simulink model "eps_tno_interface_concept"  (R2016b)
settings: Solver=FixedStepAuto  StartTime=0.0  StopTime=inf  FixedStep=0.02  RelTol=1e-3
PostLoadFcn:
  | , if any(exist('dsrtsu_mdlpostloadfcn', 'file') == [2, 3, 6]), try dsrtsu_mdlpostloadfcn('Execute', bdroot); catch fprintf('Error in PostLoadFcn (dsrtsu_mdlpostloadfcn) for model "%s":\n %s\n', bdroot, lasterr); end, end,
libraries: rtican x8, simulink x8, AlgoLib x4
(part 2 of 2)

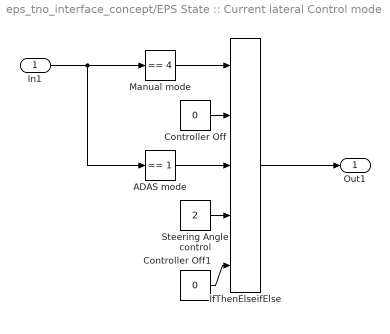
== system eps_tno_interface_concept/EPS State :: Current lateral Control mode ==
  In1 : Inport
  ADAS mode : simulink/Logic and Bit Operations/Compare To Constant  relop===  const=1  OutDataTypeStr=boolean
  Controller Off : Constant  Value=0
  Controller Off1 : Constant  Value=0
  IfThenElseifElse : AlgoLib/Signals/IfThenElseifElse
  Manual mode : simulink/Logic and Bit Operations/Compare To Constant  relop===  const=4  OutDataTypeStr=boolean
  Steering Angle control : Constant  Value=2
  Out1 : Outport
  wires:
  Controller Off1/1 -> IfThenElseifElse/5
  IfThenElseifElse/1 -> Out1/1
  Manual mode/1 -> IfThenElseifElse/1
  Controller Off/1 -> IfThenElseifElse/2
  In1/1 -> ADAS mode/1, Manual mode/1
  Steering Angle control/1 -> IfThenElseifElse/4
  ADAS mode/1 -> IfThenElseifElse/3

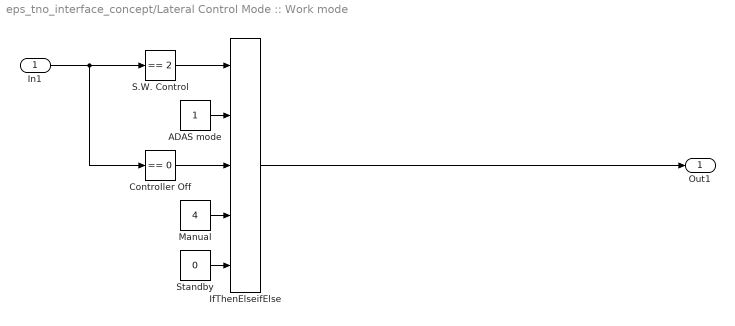
== system eps_tno_interface_concept/Lateral Control Mode :: Work mode  ==
  In1 : Inport
  ADAS mode : Constant
  Controller Off : simulink/Logic and Bit Operations/Compare To Constant  relop===  const=0  OutDataTypeStr=boolean
  IfThenElseifElse : AlgoLib/Signals/IfThenElseifElse
  Manual : Constant  Value=4
  S.W. Control : simulink/Logic and Bit Operations/Compare To Constant  relop===  const=2  OutDataTypeStr=boolean
  Standby : Constant  Value=0
  Out1 : Outport
  wires:
  Standby/1 -> IfThenElseifElse/5
  IfThenElseifElse/1 -> Out1/1
  S.W. Control/1 -> IfThenElseifElse/1
  ADAS mode/1 -> IfThenElseifElse/2
  In1/1 -> Controller Off/1, S.W. Control/1
  Manual/1 -> IfThenElseifElse/4
  Controller Off/1 -> IfThenElseifElse/3

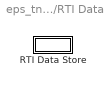
== system eps_tno_interface_concept/RTI Data ==
  RTI Data Store : Subsystem  Tag="struct('private',struct('version',struct('dsVer',uint32(2),'dsVerCreation',uint32(2),'RTI',struct('ver','7.7','type','RTI1401')),'access',struct('type','Model','isPerm',1,'created',['14-Feb-2018 14:53:06'],'modified',['03-Apr-2018 09:58:53'],'location','')),'public',struct('main',struct('data',[]),'sub',struct('name',{{'eps_tno_interfrace_concept'}},'data',{{struct('TH',struct('thTaskInfo',struct('taskType',{'TIMER','HWINT','TMRINT','SWINT','GLINT'},'tasksNumOf',{1,0,0,0,0},'srcIds',{{'TIMERA'},{},{},{},{}},'taskNames',{{['Timer Task 1']},{},{},{},{}})),'th_tc',struct('dataType','TASK','taskGroupId','','taskGroupList',{{}},'taskSchedulingPolicy','FCFS','taskType','TIMER','blkh',-1,'srcId','TIMERA','srcSgnName',['Timer A interrupt'],'srcCpuName','','taskName',['Timer Task 1  [0.02] s'],'taskNameDisplayExt','','smplTime',0.02,'smplTimeOffs',0,'hasFixedPriority',0,'priority',1,'hasFixedOvc',0,'ovcType',1,'ovcMax',1),'tc_th',struct('dataType','TASK','taskGroupId','','taskGroupList',{{}},'taskSchedulingPolicy','FCFS','taskType','TIMER','blkh',-1,'srcId','TIMERA','srcSgnName',['Timer A interrupt'],'srcCpuName','','taskName',['Timer Task 1  [0.02] s'],'taskNameDisplayExt','','smplTime',0.02,'smplTimeOffs',0,'hasFixedPriority',0,'priority',1,'hasFixedOvc',0,'ovcType',1,'ovcMax',1))}})))"  mask(RTI_DATA_STORE){}
      mask help:
      | RTI Data Store Block. This block is used by RTI to store internal model dependent data. Deleting this block will result in data loss.
      |
      | NEVER DELETE, COPY, OR MODIFY THIS BLOCK!
      mask Help:
      | RTI Data Store Block. This block is used by RTI to store internal model dependent data. Deleting this block will result in data loss.
      | 
      | NEVER DELETE, COPY, OR MODIFY THIS BLOCK!
      mask Display: text(0.5, 0.5, ' ', 'HorizontalAlignment', 'center');

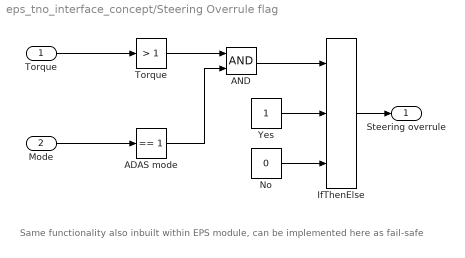
== system eps_tno_interface_concept/Steering Overrule flag ==
  note: Same functionality also inbuilt within EPS module, can be implemented here as fail-safe
  Torque : Inport
  Mode : Inport  Port=2
  ADAS mode : simulink/Logic and Bit Operations/Compare To Constant  relop===  const=1  OutDataTypeStr=boolean
  AND : Logic
  IfThenElse : AlgoLib/Signals/IfThenElse
  No : Constant  Value=0  OutDataTypeStr=boolean
  "Torque " : simulink/Logic and Bit Operations/Compare To Constant  relop=>  const=1  OutDataTypeStr=boolean
  Yes : Constant  OutDataTypeStr=boolean
  Steering overrule : Outport
  wires:
  No/1 -> IfThenElse/3
  Yes/1 -> IfThenElse/2
  Torque/1 -> "Torque "/1
  Mode/1 -> ADAS mode/1
  "Torque "/1 -> AND/1
  ADAS mode/1 -> AND/2
  AND/1 -> IfThenElse/1
  IfThenElse/1 -> Steering overrule/1

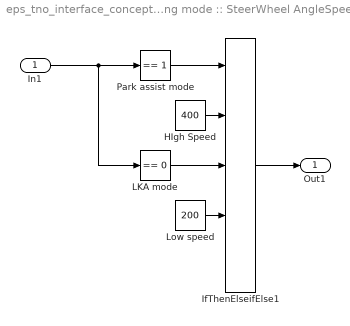
== system eps_tno_interface_concept/Steering mode :: SteerWheel AngleSpeed_ref ==
  In1 : Inport
  HIgh Speed : Constant  Value=400
  IfThenElseifElse1 : AlgoLib/Signals/IfThenElseifElse
  LKA mode : simulink/Logic and Bit Operations/Compare To Constant  relop===  const=0  OutDataTypeStr=boolean
  Low speed : Constant  Value=200
  Park assist mode : simulink/Logic and Bit Operations/Compare To Constant  relop===  const=1  OutDataTypeStr=boolean
  Out1 : Outport
  wires:
  HIgh Speed/1 -> IfThenElseifElse1/2
  Low speed/1 -> IfThenElseifElse1/4
  Park assist mode/1 -> IfThenElseifElse1/1
  LKA mode/1 -> IfThenElseifElse1/3
  IfThenElseifElse1/1 -> Out1/1
  In1/1 -> LKA mode/1, Park assist mode/1

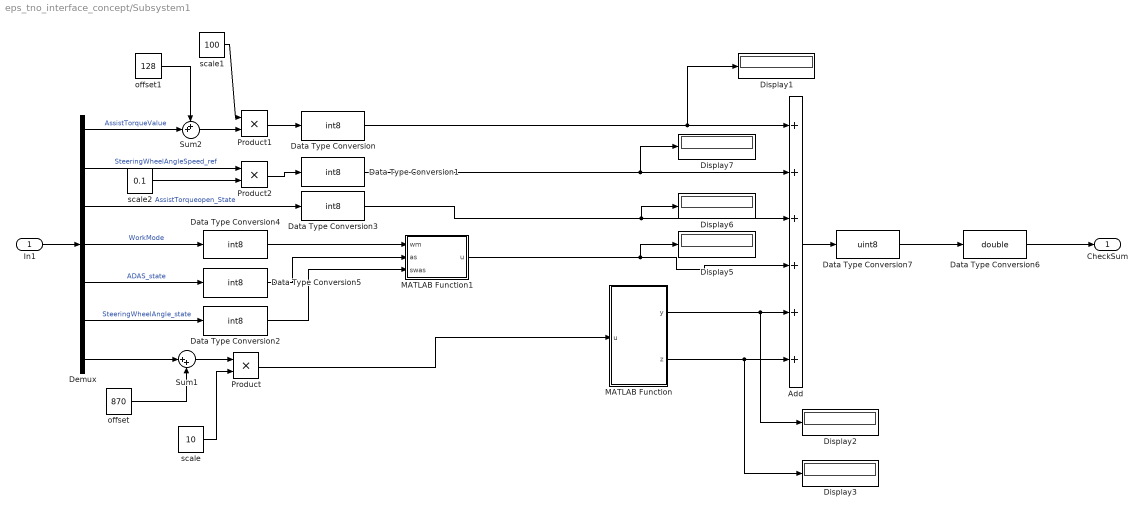
== system eps_tno_interface_concept/Subsystem1 ==
  In1 : Inport
  Add : Sum  Inputs=++++++
  Data Type Conversion{,1..5} (6 alike) : DataTypeConversion  OutDataTypeStr=int8
  Data Type Conversion6 : DataTypeConversion  OutDataTypeStr=double
  Data Type Conversion7 : DataTypeConversion  OutDataTypeStr=uint8
  Demux : Demux  Outputs=7
  Display{1..3,5..7} (6 alike) : Display
  MATLAB Function : MATLAB Function  TreatAsAtomicUnit=on
  MATLAB Function1 : MATLAB Function  TreatAsAtomicUnit=on
  Product : Product
  Product1 : Product
  Product2 : Product
  Sum1 : Sum  Inputs=|++
  Sum2 : Sum  Inputs=++|
  offset : Constant  Value=870
  offset1 : Constant  Value=128
  scale : Constant  Value=10
  scale1 : Constant  Value=100
  scale2 : Constant  Value=0.1
  CheckSum : Outport
  wires:
  In1/1 -> Demux/1
  Demux/2 -> Product2/1  "SteeringWheelAngleSpeed_ref"
  Demux/6 -> Data Type Conversion2/1  "SteeringWheelAngle_state"
  Demux/5 -> Data Type Conversion5/1  "ADAS_state"
  Demux/4 -> Data Type Conversion4/1  "WorkMode"
  Demux/3 -> Data Type Conversion3/1  "AssistTorqueopen_State"
  Data Type Conversion/1 -> Display1/1, Add/1
  Data Type Conversion1/1 -> Display7/1, Add/2
  Data Type Conversion3/1 -> Display6/1, Add/3
  Product/1 -> MATLAB Function/1(u)
  MATLAB Function/1(y) -> Display2/1, Add/5
  Data Type Conversion4/1 -> MATLAB Function1/1(wm)
  Data Type Conversion5/1 -> MATLAB Function1/2(as)
  Data Type Conversion2/1 -> MATLAB Function1/3(swas)
  MATLAB Function1/1(u) -> Display5/1, Add/4
  MATLAB Function/2(z) -> Display3/1, Add/6
  Add/1 -> Data Type Conversion7/1
  scale/1 -> Product/2
  Sum1/1 -> Product/1
  offset/1 -> Sum1/2
  Demux/7 -> Sum1/1
  Product1/1 -> Data Type Conversion/1
  Demux/1 -> Sum2/2  "AssistTorqueValue"
  offset1/1 -> Sum2/1
  scale1/1 -> Product1/1
  scale2/1 -> Product2/2
  Product2/1 -> Data Type Conversion1/1
  Sum2/1 -> Product1/2
  Data Type Conversion7/1 -> Data Type Conversion6/1
  Data Type Conversion6/1 -> CheckSum/1

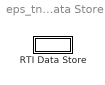
== system eps_tno_interface_concept/RTI Data/RTI Data Store ==
  RTI Data Store : Subsystem  mask(RTI_DATA_STORE){}
      mask help:
      | RTI Data Store Block. This block is used by RTI to store internal model dependent data. Deleting this block will result in data loss.
      |
      | NEVER DELETE, COPY, OR MODIFY THIS BLOCK!
      mask Help:
      | RTI Data Store Block. This block is used by RTI to store internal model dependent data. Deleting this block will result in data loss.
      | 
      | NEVER DELETE, COPY, OR MODIFY THIS BLOCK!
      mask Display: text(0.5, 0.5, ' ', 'HorizontalAlignment', 'center');

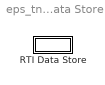
== system eps_tno_interface_concept/RTI Data/RTI Data Store/RTI Data Store ==
  RTI Data Store : Subsystem  mask(RTI_DATA_STORE){}
      mask help:
      | RTI Data Store Block. This block is used by RTI to store internal model dependent data. Deleting this block will result in data loss.
      |
      | NEVER DELETE, COPY, OR MODIFY THIS BLOCK!
      mask Help:
      | RTI Data Store Block. This block is used by RTI to store internal model dependent data. Deleting this block will result in data loss.
      | 
      | NEVER DELETE, COPY, OR MODIFY THIS BLOCK!
      mask Display: text(0.5, 0.5, ' ', 'HorizontalAlignment', 'center');

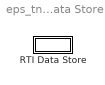
== system eps_tno_interface_concept/RTI Data/RTI Data Store/RTI Data Store/RTI Data Store ==
  RTI Data Store : Subsystem  mask(RTI_DATA_STORE){}
      mask help:
      | RTI Data Store Block. This block is used by RTI to store internal model dependent data. Deleting this block will result in data loss.
      |
      | NEVER DELETE, COPY, OR MODIFY THIS BLOCK!
      mask Help:
      | RTI Data Store Block. This block is used by RTI to store internal model dependent data. Deleting this block will result in data loss.
      | 
      | NEVER DELETE, COPY, OR MODIFY THIS BLOCK!
      mask Display: text(0.5, 0.5, ' ', 'HorizontalAlignment', 'center');

== system eps_tno_interface_concept/RTI Data/RTI Data Store/RTI Data Store/RTI Data Store/RTI Data Store ==

== matlab function eps_tno_interface_concept/Subsystem1/MATLAB Function ==
  data: u input; y output; z output
function [y, z]= fcn(u)

y=uint8(bitand(u,uint16(255)));
z=int8(bitshift(u, -8));

== matlab function eps_tno_interface_concept/Subsystem1/MATLAB Function1 ==
  data: wm input; u output; as input; swas input
function u = fcn(wm, as, swas)

assl = bitshift(as,4);
swassl = bitshift(swas, 5);

z=bitor(assl, swassl);
u=bitor(z, wm);
